simulink model "Fixed"  (R2022b)
settings: Solver=FixedStepAuto  StartTime=0.0  StopTime=20  RelTol=1e-3
settings Model: Creator=sakyu  LastModifiedBy=sakyu

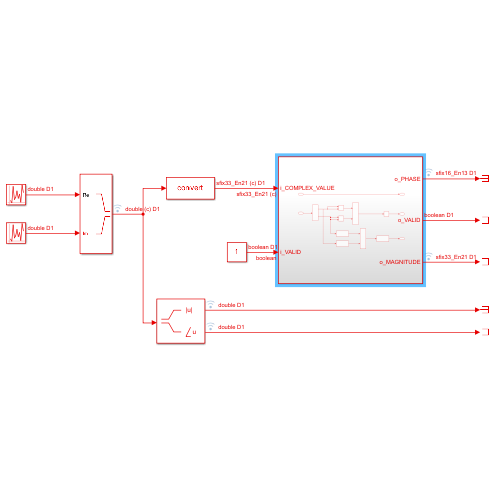
[thumbnail: Simulink's stored preview of the top-level diagram]
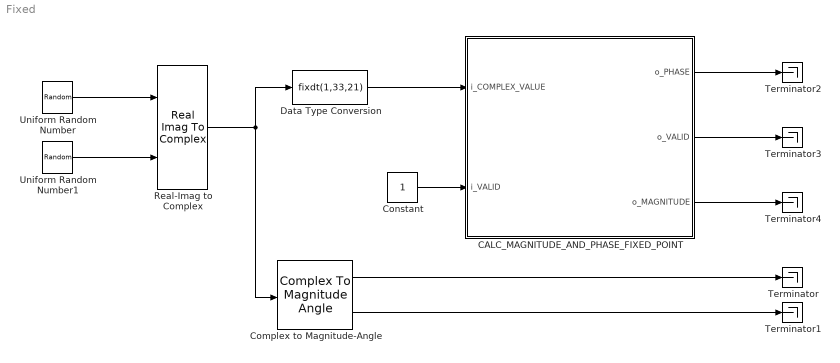
== system Fixed ==
  CALC_MAGNITUDE_AND_PHASE_FIXED_POINT : Subsystem
  Complex to Magnitude-Angle : ComplexToMagnitudeAngle
  Constant : Constant  OutDataTypeStr=boolean  SampleTime=1
  Data Type Conversion : DataTypeConversion  OutDataTypeStr=fixdt(1,33,21)  RndMeth=Round  SaturateOnIntegerOverflow=off
  Real-Imag to Complex : RealImagToComplex
  Terminator{,1..4} (5 alike) : Terminator
  Uniform Random Number : UniformRandomNumber  Minimum=0  Maximum=2047.99999904632568359375  Seed=11  SampleTime=1
  Uniform Random Number1 : UniformRandomNumber  Minimum=0  Maximum=2047.999999523162841796875  Seed=12  SampleTime=1
  wires:
  Uniform Random Number/1 -> Real-Imag to Complex/1
  Uniform Random Number1/1 -> Real-Imag to Complex/2
  Real-Imag to Complex/1 -> Complex to Magnitude-Angle/1, Data Type Conversion/1
  Complex to Magnitude-Angle/1 -> Terminator/1
  Complex to Magnitude-Angle/2 -> Terminator1/1
  Data Type Conversion/1 -> CALC_MAGNITUDE_AND_PHASE_FIXED_POINT/1(i_COMPLEX_VALUE)
  Constant/1 -> CALC_MAGNITUDE_AND_PHASE_FIXED_POINT/2(i_VALID)
  CALC_MAGNITUDE_AND_PHASE_FIXED_POINT/3(o_MAGNITUDE) -> Terminator4/1
  CALC_MAGNITUDE_AND_PHASE_FIXED_POINT/2(o_VALID) -> Terminator3/1
  CALC_MAGNITUDE_AND_PHASE_FIXED_POINT/1(o_PHASE) -> Terminator2/1

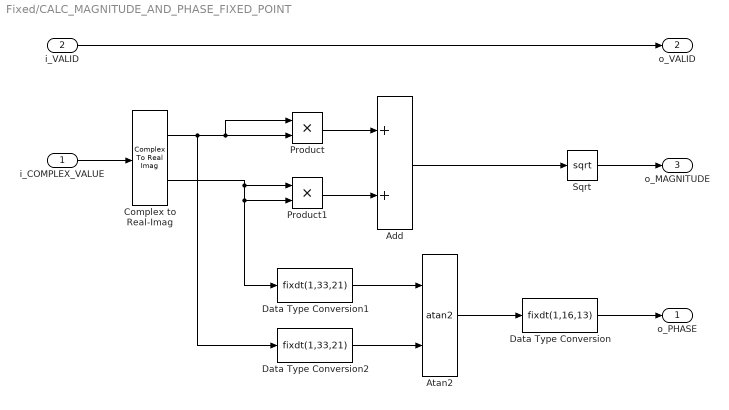
== system Fixed/CALC_MAGNITUDE_AND_PHASE_FIXED_POINT ==
  i_COMPLEX_VALUE : Inport  OutDataTypeStr=fixdt(1,33,21)
  i_VALID : Inport  Port=2  OutDataTypeStr=boolean
  Add : Sum  OutDataTypeStr=fixdt(1,66,42)
  Atan2 : Trigonometry  Operator=atan2  ApproximationMethod=CORDIC  NumberOfIterations=20
  Complex to Real-Imag : ComplexToRealImag
  Data Type Conversion : DataTypeConversion  OutDataTypeStr=fixdt(1,16,13)  SaturateOnIntegerOverflow=off  RndMeth=Floor
  Data Type Conversion1 : DataTypeConversion  OutDataTypeStr=fixdt(1,33,21)  SaturateOnIntegerOverflow=off  RndMeth=Floor
  Data Type Conversion2 : DataTypeConversion  OutDataTypeStr=fixdt(1,33,21)  SaturateOnIntegerOverflow=off  RndMeth=Floor
  Product : Product  OutDataTypeStr=fixdt(1,65,42)
  Product1 : Product  OutDataTypeStr=fixdt(1,65,42)
  Sqrt : Sqrt  OutDataTypeStr=fixdt(1,33,21)
  o_PHASE : Outport
  o_VALID : Outport  Port=2
  o_MAGNITUDE : Outport  Port=3
  wires:
  Complex to Real-Imag/2 -> Data Type Conversion1/1, Product1/2, Product1/1
  Product/1 -> Add/1
  Product1/1 -> Add/2
  Complex to Real-Imag/1 -> Data Type Conversion2/1, Product/1, Product/2
  Add/1 -> Sqrt/1
  Atan2/1 -> Data Type Conversion/1
  i_VALID/1 -> o_VALID/1
  Sqrt/1 -> o_MAGNITUDE/1
  Data Type Conversion/1 -> o_PHASE/1
  Data Type Conversion1/1 -> Atan2/1
  Data Type Conversion2/1 -> Atan2/2
  i_COMPLEX_VALUE/1 -> Complex to Real-Imag/1
